simulink model "signal_generator"  (R2020a)
settings: Solver=VariableStepAuto  StartTime=0.0  StopTime=4  RelTol=1e-3
settings Model: Creator=HP  LastModifiedBy=HP

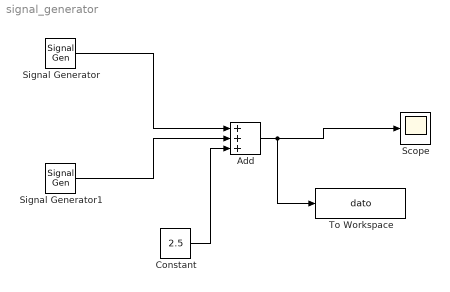
== system signal_generator ==
  Add : Sum  Inputs=+++
  Constant : Constant  Value=2.5
  Scope : Scope
  Signal Generator : SignalGenerator  Amplitude=2  Frequency=0.5
  Signal Generator1 : SignalGenerator  Amplitude=0.5  Frequency=80  Units=rad/sec
  To Workspace : ToWorkspace  VariableName=dato  SampleTime=-1
      settings: Save2DSignal=2-D array (concatenate along first dimension)
  wires:
  Add/1 -> To Workspace/1, Scope/1
  Signal Generator1/1 -> Add/2
  Signal Generator/1 -> Add/1
  Constant/1 -> Add/3
